simulink model "W04_S1"  (R2024b)
settings: Solver=ode4  StartTime=0  StopTime=T_final  FixedStep=h  RelTol=1e-3
values from neighbouring files (symbols this model uses):
  x0 = zeros(12,1); x0(12) = deg2rad(170)    [W04_S_expected.m]
undefined symbols (not defined in the file or in its folder): beta_c, k_neg, k_pos, Kd, Ki, Kp, mp, n_max, n_min, Nf, psi_step, rp, t_step, use_ssa, V_c, X_ff, y_pont
settings Model: Creator=admin  LastModifiedBy=admin
settings DataIOCC: ReturnWorkspaceOutputs=off

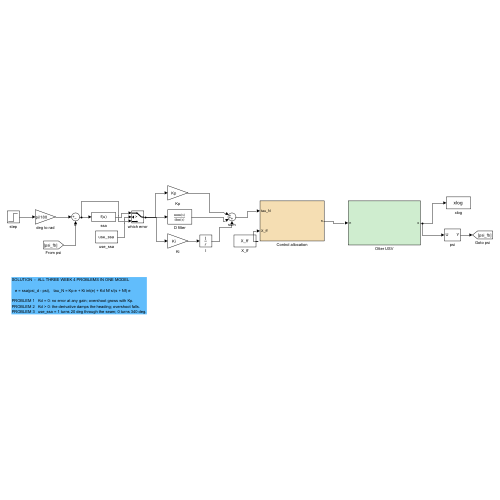
[thumbnail: Simulink's stored preview of the top-level diagram]
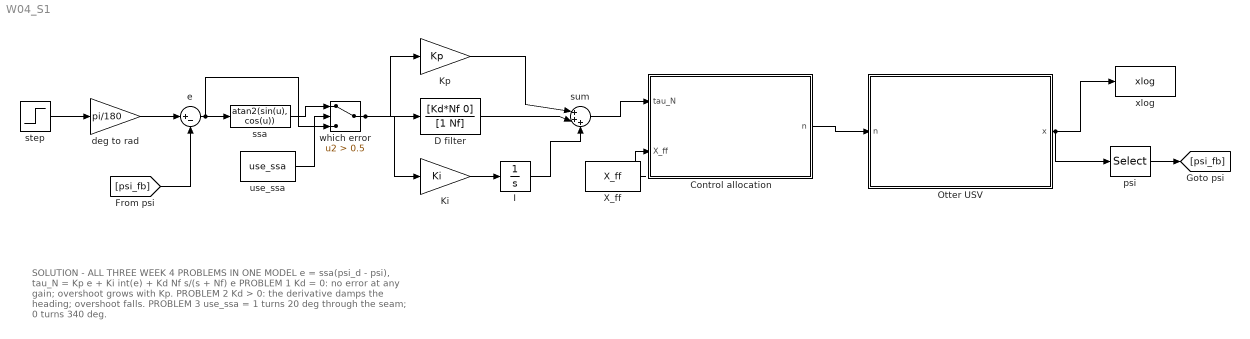
== system W04_S1 ==
  note: SOLUTION  -  ALL THREE WEEK 4 PROBLEMS IN ONE MODEL
      |
      |    e = ssa(psi_d - psi),   tau_N = Kp e + Ki int(e) + Kd Nf s/(s + Nf) e
      |
      | PROBLEM 1   Kd = 0: no error at any gain; overshoot grows with Kp.
      | PROBLEM 2   Kd > 0: the derivative damps the heading; overshoot falls.
      | PROBLEM 3   use_ssa = 1 turns 20 deg through the seam; 0 turns 340 deg.
  Control allocation : Subsystem
  D filter : TransferFcn  Numerator=[Kd*Nf 0]  Denominator=[1 Nf]
  I : Integrator
  Ki : Gain  Gain=Ki
  Kp : Gain  Gain=Kp
  Otter USV : Subsystem
  X_ff : Constant  Value=X_ff
  deg to rad : Gain  Gain=pi/180
  e : Sum  Inputs=|+-
  psi : Selector  InputPortWidth=12  IndexOptions=Index vector (dialog)  Indices=12  OutputSizes=1
  ssa : Fcn  Expr=atan2(sin(u), cos(u))
  step : Step  Time=t_step  After=psi_step  SampleTime=0
  sum : Sum  Inputs=|+++
  use_ssa : Constant  Value=use_ssa
  which error : Switch  Criteria=u2 > Threshold  Threshold=0.5  SaturateOnIntegerOverflow=off  InputSameDT=off
  xlog : ToWorkspace  VariableName=xlog  SaveFormat=Structure With Time  SampleTime=-1
  wires:
  step/1 -> deg to rad/1
  deg to rad/1 -> e/1
  e/1 -> ssa/1, which error/3
  ssa/1 -> which error/1
  use_ssa/1 -> which error/2
  which error/1 -> Kp/1, D filter/1, Ki/1
  Ki/1 -> I/1
  Kp/1 -> sum/1
  D filter/1 -> sum/2
  I/1 -> sum/3
  sum/1 -> Control allocation/1(tau_N)
  X_ff/1 -> Control allocation/2(X_ff)
  Control allocation/1(n) -> Otter USV/1(n)
  Otter USV/1(x) -> xlog/1, psi/1
  psi/1 -> [psi_fb]
  [psi_fb] -> e/2

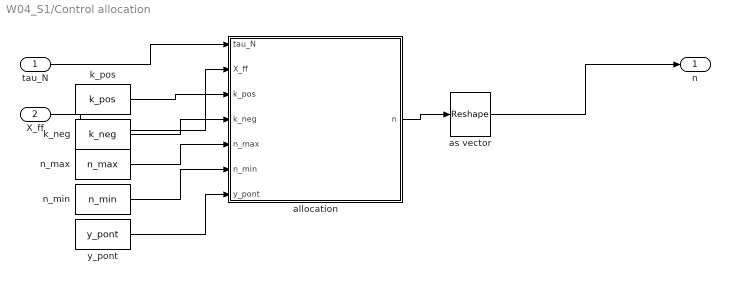
== system W04_S1/Control allocation ==
  tau_N : Inport
  X_ff : Inport  Port=2
  allocation : MATLAB Function  TreatAsAtomicUnit=on
  as vector : Reshape
  k_neg : Constant  Value=k_neg
  k_pos : Constant  Value=k_pos
  n_max : Constant  Value=n_max
  n_min : Constant  Value=n_min
  y_pont : Constant  Value=y_pont
  n : Outport
  wires:
  k_pos/1 -> allocation/3(k_pos)
  k_neg/1 -> allocation/4(k_neg)
  n_max/1 -> allocation/5(n_max)
  n_min/1 -> allocation/6(n_min)
  y_pont/1 -> allocation/7(y_pont)
  tau_N/1 -> allocation/1(tau_N)
  X_ff/1 -> allocation/2(X_ff)
  allocation/1(n) -> as vector/1
  as vector/1 -> n/1

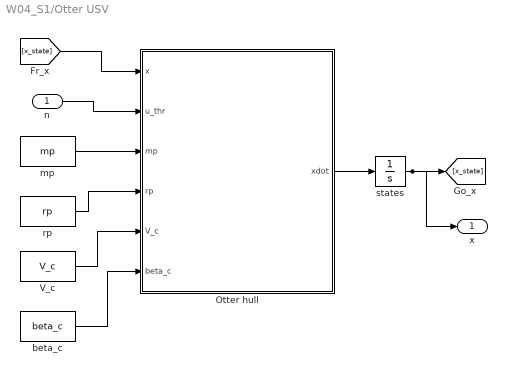
== system W04_S1/Otter USV ==
  n : Inport
  Otter hull : MATLAB Function  TreatAsAtomicUnit=on
  V_c : Constant  Value=V_c
  beta_c : Constant  Value=beta_c
  mp : Constant  Value=mp
  rp : Constant  Value=rp
  states : Integrator  InitialCondition=x0
  x : Outport
  wires:
  states/1 -> [x_state], x/1
  [x_state] -> Otter hull/1(x)
  Otter hull/1(xdot) -> states/1
  beta_c/1 -> Otter hull/6(beta_c)
  V_c/1 -> Otter hull/5(V_c)
  rp/1 -> Otter hull/4(rp)
  mp/1 -> Otter hull/3(mp)
  n/1 -> Otter hull/2(u_thr)

== matlab function W04_S1/Otter USV/Otter hull ==
  data: x input; xdot output double size=[12 1]; u_thr input; mp input; rp input; V_c input; beta_c input
function xdot = otter_hull(x, u_thr, mp, rp, V_c, beta_c)
% Fossen's otter.m, called unchanged from Tools/MSS/VESSELS.
%
%   x       12 states, fed back from the integrator
%   u_thr   propeller shaft speeds [rad/s]
%
% otter.m is not written for code generation, so the call is extrinsic and
% xdot has to be pre-sized for Simulink to know the output width.
coder.extrinsic('otter');

xdot = zeros(12,1);
xdot = otter(x, u_thr, mp, rp, V_c, beta_c);
end

== matlab function W04_S1/Control allocation/allocation ==
  data: tau_N input; n output double size=[2 1]; X_ff input; k_pos input; k_neg input; n_max input; n_min input; y_pont input
function n = allocation(tau_N, X_ff, k_pos, k_neg, n_max, n_min, y_pont)
%#codegen
% Demanded surge force and yaw moment to two shaft speeds.
T = [X_ff/2 + tau_N/(2*y_pont);
     X_ff/2 - tau_N/(2*y_pont)];
n = zeros(2,1);
for i = 1:2
    if T(i) >= 0
        ni =  sqrt( T(i) / k_pos);
    else
        ni = -sqrt(-T(i) / k_neg);
    end
    n(i) = min(max(ni, n_min), n_max);
end
end
